simulink model "bus_roadtest_v3"  (R2018a)
settings: Solver=ode3  StartTime=0.0  StopTime=inf  FixedStep=0.01  RelTol=1e-3  EnableMultiTasking=on
PostLoadFcn:
  | , if any(exist('dsrtsu_mdlpostloadfcn', 'file') == [2, 3, 6]), try dsrtsu_mdlpostloadfcn('Execute', bdroot); catch fprintf('Error in PostLoadFcn (dsrtsu_mdlpostloadfcn) for model "%s":\n %s\n', bdroot, lasterr); end, end,
InitFcn:
  | bus_roadtest_v3_initial
values from neighbouring files (symbols this model uses):
  ay_max = 2    [Ini.m]
  delta_t = 0.01    [Ini.m]
  end_left_pass = 1    [Ini.m]
  end_right_pass = 0    [Ini.m]
  finish_node_id = length(Map_data(:,1))    [Ini.m]
  forward_length = 15    [Ini.m]
  gamma = sqrt(N_xaug+lambda)    [bus_roadtest_v3_initial.m]
  k_safe = 1    [Ini.m]
  nodes = nodes(1:index_node,:)    [Ini.m]
  rmin = 10    [Ini.m]
  segments = zeros(length(xy_ends_Pos(:,1)),3)    [Ini.m]
  start_node_id = 1    [Ini.m]
  Ts = 0.01    [bus_roadtest_v3_initial.m]
  Veh_CG = [0.5, 0.2]    [Ini.m]
  Veh_size = [1.99986,6.09558]    [Ini.m]
  vmax = 6    [Ini.m]
  weight = [weight_0,weight_0_cov,weight_i]    [bus_roadtest_v3_initial.m]
undefined symbols (not defined in the file or in its folder): Brake_table, DiscIntNeverNeededParam, Map_data, R, REF_GPS_RFS, Steer_gain_table, T
libraries: rtican x71, simulink x26, rti1401lib_adc_type4 x8, rti1401lib_dio_type4 x1
(part 10 of 18)

== system bus_roadtest_v3/Flag_management/Button management ==
  Button management : MATLAB Function  TreatAsAtomicUnit=on
  Delay3 : Delay  DelayLength=1  InitialCondition=0
  "[Disp] Door1_close_button" : Display
  "[Disp] Door1_open_button" : Display
  "[Disp] Door2_button" : Display
  "[Disp] Door_cmd" : Display
  "[Disp] Door_switch_button" : Display
  "[Disp] Drive_start" : Display
  "[Disp] Drive_start_button" : Display
  "[Disp] Drive_stop" : Display
  "[Disp] Drive_stop_button" : Display
  "[Disp] Emergency_button" : Display
  "[Disp] Emergency_stop" : Display
  "[Disp] PLC_door" : Display
  Drive_start : Outport
  Drive_stop : Outport  Port=2
  Emergency_stop : Outport  Port=3
  Door_cmd : Outport  Port=4
  wires:
  Button management/2(Drive_stop) -> Drive_stop/1, "[Disp] Drive_stop"/1
  Delay3/1 -> Button management/9(Auto_Door)
  Button management/3(Emergency_stop) -> Emergency_stop/1, "[Disp] Emergency_stop"/1
  [Drive_start_button] -> "[Disp] Drive_start_button"/1, Button management/1(Drive_start_button)
  [Door1_open_button] -> "[Disp] Door1_open_button"/1, Button management/5(Door1_open_button)
  Button management/1(Drive_start) -> Drive_start/1, "[Disp] Drive_start"/1
  [Auto_Door] -> Delay3/1
  [Drive_stop_button] -> "[Disp] Drive_stop_button"/1, Button management/2(Drive_stop_button)
  [Door1_close_button] -> "[Disp] Door1_close_button"/1, Button management/6(Door1_close_button)
  [PLC_door] -> "[Disp] PLC_door"/1, Button management/4(Door_state_fb)
  [Emergency_button] -> "[Disp] Emergency_button"/1, Button management/3(Emergency_button)
  [Door_switch_button] -> "[Disp] Door_switch_button"/1, Button management/8(Door_switch_button)
  [Door2_button] -> "[Disp] Door2_button"/1, Button management/7(Door2_button)
  Button management/4(Door_cmd) -> Door_cmd/1, "[Disp] Door_cmd"/1

== system bus_roadtest_v3/Flag_management/Fault detection ==
  Fault detection(Control) : Subsystem
  Fault flags management : MATLAB Function  TreatAsAtomicUnit=on
  "[Disp] Fault_minor" : Display
  "[Disp] Fault_prime" : Display
  Fault_minor : Outport
  Fault_prime : Outport  Port=2
  tag scope: Brake_fault=global, Localization_fault=global, OBU_fault=global, RSU_fault=global, Speed_fault=global, Steer_fault=global
  wires:
  [SLAM_fault] -> Fault flags management/7(SLAM_fault)
  [Speed_fault] -> Fault flags management/3(Speed_fault)
  [OBU_fault] -> Fault flags management/2(OBU_fault)
  [Monitor_fault] -> Fault flags management/1(Monitor_fault)
  [Steer_fault] -> Fault flags management/4(Steer_fault)
  [Brake_fault] -> Fault flags management/5(Brake_fault)
  [RSU_fault] -> Fault flags management/6(RSU_fault)
  Fault detection(Control)/1(Speed_fault) -> [Speed_fault]
  Fault detection(Control)/6(OBU_fault) -> [OBU_fault]
  Fault detection(Control)/5(RSU_fault) -> [RSU_fault]
  Fault detection(Control)/4(SLAM_fault) -> [Localization_fault]
  Fault detection(Control)/3(Brake_fault) -> [Brake_fault]
  Fault detection(Control)/2(Steer_fault) -> [Steer_fault]
  Fault flags management/2(Fault_prime) -> Fault_prime/1, "[Disp] Fault_prime"/1
  Fault flags management/1(Fault_minor) -> Fault_minor/1, "[Disp] Fault_minor"/1

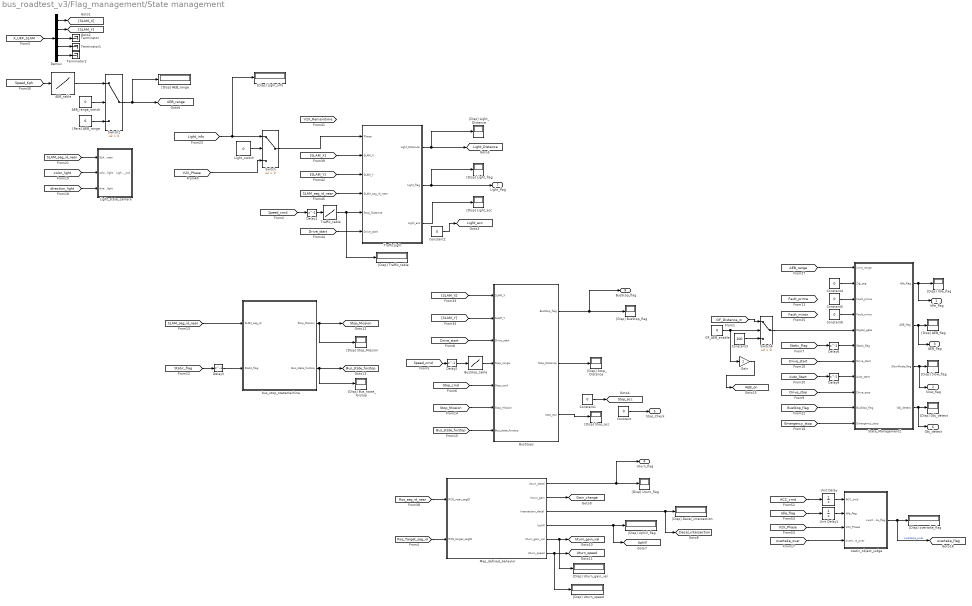
== system bus_roadtest_v3/Flag_management/State management ==
  " BusStops" : MATLAB Function  TreatAsAtomicUnit=on
  AEB_range_switch : Constant  Value=0
  AEB_table : Lookup_n-D  NumberOfTableDimensions=1  BreakpointsForDimension1="[0 5 10 15  20]"  Table=[3 3 4 6 8]  InternalRulePriority=Speed  RndMeth=Simplest  InputSameDT=on
  BusStop_table : Lookup_n-D  NumberOfTableDimensions=1  BreakpointsForDimension1=[0 5 9 13 17]  Table=[4 5.5 11 17 25]  InternalRulePriority=Speed  RndMeth=Simplest  InputSameDT=on
  Constant{,1..2,4..6} (6 alike) : Constant  Value=0
  Constant3 : Constant  Value=100
  Delay{1..3,6,9} (5 alike) : Delay  DelayLength=1  InitialCondition=0
  Demux : Demux  Outputs=5
  GF_AEB_enable : Constant  Value=0
  Gain : Gain
  "Light_state_camera " : MATLAB Function  TreatAsAtomicUnit=on
  Light_switch : Constant  Value=0  VectorParams1D=off  SampleTime=-1
  Map_defined_behavior : MATLAB Function  TreatAsAtomicUnit=on
  State_Management2 : MATLAB Function  TreatAsAtomicUnit=on
  Switch : Switch  Criteria=u2 > Threshold
  Switch2 : Switch  Criteria=u2 > Threshold
  Switch6 : Switch  Criteria=u2 > Threshold
  Terminator : Terminator
  Terminator1 : Terminator
  Terminator2 : Terminator
  TrafficLight : MATLAB Function  TreatAsAtomicUnit=on
  Traffic_table : Lookup_n-D  NumberOfTableDimensions=1  BreakpointsForDimension1=[0 5 9 13 17]  Table=[4 5.5 11 16.5 25]  InternalRulePriority=Speed  RndMeth=Simplest  InputSameDT=on
  Unit Delay : UnitDelay  SampleTime=-1
  Unit Delay1 : UnitDelay  SampleTime=-1
  "[Disp] AEB_flag" : Display
  "[Disp] AEB_range" : Display
  "[Disp] BusStop_flag" : Display
  "[Disp] Bus_state_forstop" : Display
  "[Disp] Decel_intersection" : Display
  "[Disp] Idle_flag" : Display
  "[Disp] Light_Distance" : Display
  "[Disp] Light_acc" : Display
  "[Disp] Light_flag" : Display
  "[Disp] Light_info" : Display
  "[Disp] Obj_detect" : Display
  "[Disp] Slow_flag" : Display
  "[Disp] Stop_Distance" : Display
  "[Disp] Stop_Mission" : Display
  "[Disp] Stop_acc" : Display
  "[Disp] Traffic_table" : Display
  "[Disp] Uphill_flag" : Display
  "[Disp] Uturn_flag" : Display
  "[Disp] Uturn_gain_val" : Display
  "[Disp] Uturn_speed" : Display
  "[Disp] overtake_flag" : Display
  "[Para] AEB_range" : Constant  Value=6
  bus_stop_statemachine : MATLAB Function  TreatAsAtomicUnit=on
  static_object_judge : MATLAB Function  TreatAsAtomicUnit=on
  Idle_flag : Outport
  Slow_flag : Outport  Port=2
  AEB_flag : Outport  Port=3
  Uturn_flag : Outport  Port=4
  Stop_Check : Outport  Port=5
  Obj_detect : Outport  Port=6
  Light_flag : Outport  Port=7
  BusStop_flag : Outport  Port=8
  tag scope: AEB_on=global, AEB_range=global, Bus_state_forstop=global, Decel_intersection=global, Gain_change=global, Light_Distance=global, Light_acc=global, Stop_Mission=global, Stop_acc=global, Uphill=global, Uturn_gain_val=global, Uturn_speed=global, overtake_flag=global
  wires:
  [Static_flag] -> Delay6/1
  Delay6/1 -> State_Management2/6(Static_flag)
  [Drive_stop] -> State_Management2/9(Drive_stop)
  [Drive_start] -> State_Management2/7(Drive_start)
  AEB_table/1 -> Switch2/1
  AEB_range_switch/1 -> Switch2/2
  [Speed_Kph] -> AEB_table/1
  "[Para] AEB_range"/1 -> Switch2/3
  Switch2/1 -> "[Disp] AEB_range"/1, [AEB_range]
  [AEB_range] -> State_Management2/1(Limit_range)
  [X_UKF_SLAM] -> Demux/1
  Demux/5 -> Terminator2/1
  Demux/4 -> Terminator1/1
  Demux/3 -> Terminator/1
  Demux/1 -> [SLAM_X]
  Demux/2 -> [SLAM_Y]
  [SLAM_X] -> " BusStops"/1(SLAM_X)
  [SLAM_Y] -> " BusStops"/2(SLAM_Y)
  [Ros_seg_id_near] -> Map_defined_behavior/1(ROS_near_segID)
  [Drive_start] -> " BusStops"/3(Drive_start)
  [BusStop_flag] -> State_Management2/10(BusStop_flag)
  [SLAM_Y] -> TrafficLight/3(SLAM_Y)
  [SLAM_X] -> TrafficLight/2(SLAM_X)
  [Drive_start] -> TrafficLight/6(Drive_start)
  Map_defined_behavior/1(Uturn_decel) -> Uturn_flag/1, "[Disp] Uturn_flag"/1
  State_Management2/2(AEB_flag) -> AEB_flag/1, "[Disp] AEB_flag"/1
  State_Management2/1(Idle_flag) -> Idle_flag/1, "[Disp] Idle_flag"/1
  State_Management2/4(Obj_detect) -> Obj_detect/1, "[Disp] Obj_detect"/1
  " BusStops"/2(Stop_Distance) -> "[Disp] Stop_Distance"/1
  [SLAM_seg_id_near] -> TrafficLight/4(SLAM_seg_id_near)
  [Auto_Start] -> Delay9/1
  Delay9/1 -> State_Management2/8(Auto_start)
  Constant3/1 -> Switch6/3
  Switch6/1 -> State_Management2/5(Digital_gate)
  GF_AEB_enable/1 -> Gain/1, Switch6/2
  Constant4/1 -> State_Management2/2(Zig_zag)
  Constant5/1 -> State_Management2/3(Fault_prime)
  Constant6/1 -> State_Management2/4(Fault_minor)
  State_Management2/3(SlowMode_flag) -> Slow_flag/1, "[Disp] Slow_flag"/1
  [Emergency_stop] -> State_Management2/11(Emergency_stop)
  TrafficLight/1(Light_Distance) -> "[Disp] Light_Distance"/1, [Light_Distance]
  TrafficLight/2(Light_flag) -> "[Disp] Light_flag"/1, Light_flag/1
  TrafficLight/3(Light_acc) -> "[Disp] Light_acc"/1
  [GF_Distance_m] -> Switch6/1
  [Speed_cmd] -> Delay1/1
  [Ros_Target_seg_id] -> Map_defined_behavior/2(ROS_target_segID)
  Map_defined_behavior/4(Uphill) -> "[Disp] Uphill_flag"/1, [Uphill]
  Map_defined_behavior/3(Intersection_decel) -> [Decel_intersection], "[Disp] Decel_intersection"/1
  Map_defined_behavior/2(Uturn_gain) -> [Gain_change]
  Map_defined_behavior/5(Uturn_gain_val) -> "[Disp] Uturn_gain_val"/1, [Uturn_gain_val]
  Map_defined_behavior/6(Uturn_speed) -> "[Disp] Uturn_speed"/1, [Uturn_speed]
  BusStop_table/1 -> " BusStops"/4(Stop_range)
  [Speed_cmd] -> Delay2/1
  Delay2/1 -> BusStop_table/1
  [Stop_cmd] -> " BusStops"/5(Stop_cmd)
  Delay3/1 -> bus_stop_statemachine/2(Static_flag)
  [Static_flag] -> Delay3/1
  [SLAM_seg_id_near] -> bus_stop_statemachine/1(SLAM_seg_id)
  bus_stop_statemachine/1(Stop_Mission) -> "[Disp] Stop_Mission"/1, [Stop_Mission]
  bus_stop_statemachine/2(Bus_state_forstop) -> "[Disp] Bus_state_forstop"/1, [Bus_state_forstop]
  [Stop_Mission] -> " BusStops"/6(Stop_Mission)
  [Bus_state_forstop] -> " BusStops"/7(Bus_state_forstop)
  Constant/1 -> Stop_Check/1
  " BusStops"/3(stop_acc) -> "[Disp] Stop_acc"/1
  [V2X_Phase] -> static_object_judge/3(V2X_Phase)
  [ACC_cmd] -> Unit Delay/1
  Unit Delay/1 -> static_object_judge/1(ACC_cmd)
  Unit Delay1/1 -> static_object_judge/2(Idle_flag)
  [Idle_flag] -> Unit Delay1/1
  [overtake_over] -> static_object_judge/4(overtake_over)
  Gain/1 -> [AEB_on]
  [color_light] -> "Light_state_camera "/2(color_light)
  [direction_light] -> "Light_state_camera "/3(direction_light)
  [SLAM_seg_id_near] -> "Light_state_camera "/1(SLAM_seg_id_near)
  Light_switch/1 -> Switch/2
  Switch/1 -> TrafficLight/1(Phase)
  [Light_info] -> "[Disp] Light_info"/1, Switch/1
  Delay1/1 -> Traffic_table/1
  Traffic_table/1 -> "[Disp] Traffic_table"/1, TrafficLight/5(Stop_Distance)
  [V2X_Phase] -> Switch/3
  " BusStops"/1(BusStop_flag) -> BusStop_flag/1, "[Disp] BusStop_flag"/1
  Constant1/1 -> [Stop_acc]
  Constant2/1 -> [Light_acc]
  static_object_judge/1(overtake_flag) -> [overtake_flag], "[Disp] overtake_flag"/1  "overtake_over"

== system bus_roadtest_v3/Motion_controller/Lateral_control ==
  Auto_Uturn : Constant
  Gain : Gain  Gain=-180/pi
  Gain1 : Gain  Gain=-1
  LKC_module : Subsystem
  Signal_switch1 : Switch  Criteria=u2 > Threshold
  Signal_switch2 : Switch  Criteria=u2 > Threshold
  Signal_switch3 : Switch  Criteria=u2 > Threshold
  U-turn : Constant  Value=0
  "[Disp] Angle_cmd" : Display
  "[Disp] Auto_Uturn_flag" : Display
  "[Disp] Theta_err" : Display
  "[Disp] Theta_prediction" : Display
  "[Disp] Theta_target" : Display
  "[Para] Look_ahead_Uturn" : Constant  Value=1.6
  "[Para] Look_ahead_time" : Constant  Value=1.6
  tag scope: Steer_cmd=global, U_turn=global
  wires:
  [SBG_Gyro_Z] -> Gain/1
  LKC_module/2(Theta_prediction) -> "[Disp] Theta_prediction"/1
  LKC_module/3(Theta_err) -> "[Disp] Theta_err"/1
  LKC_module/4(Theta_target) -> "[Disp] Theta_target"/1
  [Speed_mps] -> LKC_module/3(Vx)
  LKC_module/1(Steerwheel_cmd) -> [Steer_cmd], "[Disp] Angle_cmd"/1
  [Look_ahead_S0] -> LKC_module/2(Look_ahead_S0)
  Signal_switch1/1 -> LKC_module/1(Look_ahead_time)
  "[Para] Look_ahead_time"/1 -> Signal_switch1/3
  "[Para] Look_ahead_Uturn"/1 -> Signal_switch1/1
  Signal_switch2/1 -> Signal_switch1/2, [U_turn]
  U-turn/1 -> Signal_switch2/3
  Auto_Uturn/1 -> Signal_switch2/2
  [angular_vz] -> Gain1/1
  Gain1/1 -> LKC_module/5(yaw_rate_IMU)
  [Gain_change] -> "[Disp] Auto_Uturn_flag"/1, Signal_switch3/2, Signal_switch2/1
  Signal_switch3/1 -> LKC_module/4(Y_target)
  [Ros_rear_Vehicle_Target_y] -> Signal_switch3/3
  [Ros_Vehicle_Target_y] -> Signal_switch3/1

== system bus_roadtest_v3/Motion_controller/Longitudinal_control ==
  Speed_profile : Inport
  AEB_trig : Inport  Port=2
  Static : Inport  Port=3
  Brake_controller : Subsystem
  Data Type Conversion : DataTypeConversion  OutDataTypeStr=boolean
  Fbrake_Pcmd : Constant  Value=0
  Fbrake_mode : Constant
  Memory : Memory
  Rbrake_Pcmd : Constant  Value=0
  Rbrake_mode : Constant
  Switching_module : Subsystem
  Throttle_controller : Subsystem
  Throttle_mode : Constant
  Throttle_vol : Constant  Value=0
  "[Disp] Fbrake_Vcmd" : Display
  "[Disp] Rbrake_Vcmd" : Display
  "[Disp] Throttle_Vcmd" : Display
  tag scope: Fbrake_Vcmd=global, Rbrake_Vcmd=global, Throttle_Vcmd=global
  wires:
  Speed_profile/1 -> Brake_controller/9(Speed_profile), Switching_module/3(Speed_profile)
  Switching_module/3(Brake_trig_CC) -> Memory/1, Brake_controller/8(Brake_trig_CC)
  Memory/1 -> Data Type Conversion/1
  Throttle_mode/1 -> Throttle_controller/1(Throttle_mode)
  Throttle_vol/1 -> Throttle_controller/2(Throttle_vol)
  Throttle_controller/1(Throttle_out) -> "[Disp] Throttle_Vcmd"/1, [Throttle_Vcmd]
  AEB_trig/1 -> Switching_module/1(AEB_trig), Brake_controller/1(AEB_trig), Throttle_controller/3(AEB_trig)
  Static/1 -> Switching_module/2(Static), Brake_controller/2(Static), Throttle_controller/4(Static)
  Fbrake_mode/1 -> Brake_controller/4(Fbrake_mode)
  Fbrake_Pcmd/1 -> Brake_controller/5(Fbrake_Pcmd)
  Brake_controller/1(Fbrake_Vcmd) -> "[Disp] Fbrake_Vcmd"/1, [Fbrake_Vcmd]
  Data Type Conversion/1 -> Switching_module/4(Brake_trig_CC_status)
  Switching_module/1(Speed_cmd) -> Throttle_controller/5(Speed_cmd)
  Switching_module/2(Decel_cmd) -> Brake_controller/3(Decel_cmd)
  Rbrake_Pcmd/1 -> Brake_controller/7(Rbrake_Pcmd)
  Rbrake_mode/1 -> Brake_controller/6(Rbrake_mode)
  Brake_controller/2(Rbrake_Vcmd) -> "[Disp] Rbrake_Vcmd"/1, [Rbrake_Vcmd]

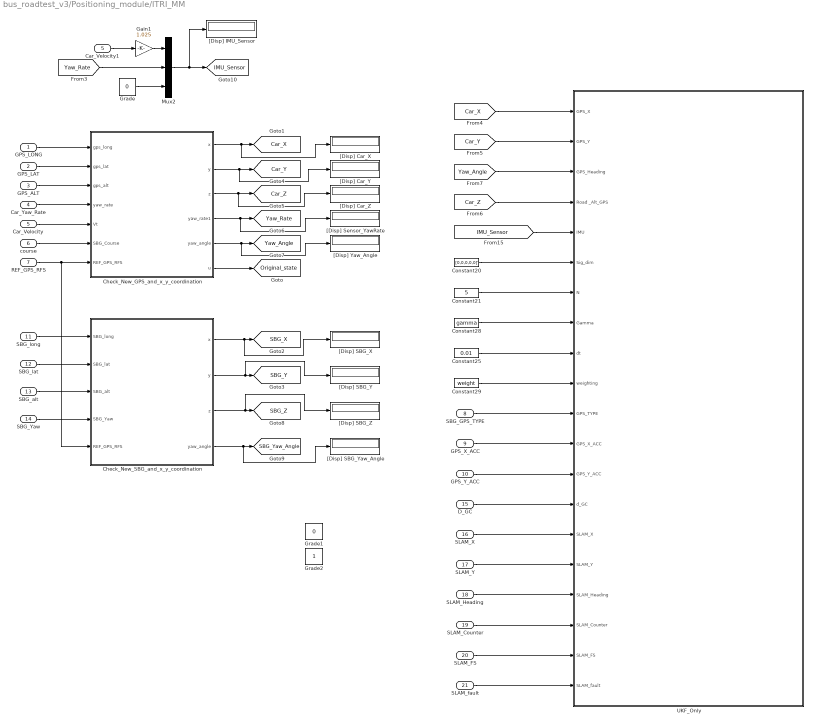
== system bus_roadtest_v3/Positioning_module/ITRI_MM ==
  GPS_LONG : Inport
  GPS_LAT : Inport  Port=2
  GPS_ALT : Inport  Port=3
  Car_Yaw_Rate : Inport  Port=4
  Car_Velocity : Inport  Port=5
  course : Inport  Port=6
  REF_GPS_RFS : Inport  Port=7
  SBG_GPS_TYPE : Inport  Port=8
  GPS_X_ACC : Inport  Port=9
  GPS_Y_ACC : Inport  Port=10
  SBG_long : Inport  Port=11
  SBG_lat : Inport  Port=12
  SBG_alt : Inport  Port=13
  SBG_Yaw : Inport  Port=14
  D_GC : Inport  Port=15
  SLAM_X : Inport  Port=16
  SLAM_Y : Inport  Port=17
  SLAM_Heading : Inport  Port=18
  SLAM_Counter : Inport  Port=19
  SLAM_FS : Inport  Port=20
  SLAM_fault : Inport  Port=21
  Car_Velocity1 : InportShadow  Port=5
  Check_New_GPS_and_x_y_coordination : MATLAB Function  TreatAsAtomicUnit=on
  Check_New_SBG_and_x_y_coordination : MATLAB Function  TreatAsAtomicUnit=on
  Constant20 : Constant  Value=[0,0,0,0,0]'
  Constant21 : Constant  Value=5
  Constant25 : Constant  Value=0.01
  Constant28 : Constant  Value=gamma
  Constant29 : Constant  Value=weight
  Gain1 : Gain  Gain=1.025
  Grade : Constant  Value=0
  Grade1 : Constant  Value=0
  Grade2 : Constant
  Mux2 : Mux  Inputs=3
  UKF_Only : Subsystem
  "[Disp] Car_X" : Display
  "[Disp] Car_Y" : Display
  "[Disp] Car_Z" : Display
  "[Disp] IMU_Sensor" : Display
  "[Disp] SBG_X" : Display
  "[Disp] SBG_Y" : Display
  "[Disp] SBG_Yaw_Angle" : Display
  "[Disp] SBG_Z" : Display
  "[Disp] Sensor_YawRate" : Display
  "[Disp] Yaw_Angle" : Display
  tag scope: Car_X=global, Car_Y=global, Car_Z=global, IMU_Sensor=global, Original_state=global, SBG_X=global, SBG_Y=global, SBG_Yaw_Angle=global, SBG_Z=global, Yaw_Angle=global, Yaw_Rate=global
  wires:
  GPS_LONG/1 -> Check_New_GPS_and_x_y_coordination/1(gps_long)
  GPS_LAT/1 -> Check_New_GPS_and_x_y_coordination/2(gps_lat)
  GPS_ALT/1 -> Check_New_GPS_and_x_y_coordination/3(gps_alt)
  Car_Yaw_Rate/1 -> Check_New_GPS_and_x_y_coordination/4(yaw_rate)
  Car_Velocity/1 -> Check_New_GPS_and_x_y_coordination/5(Vt)
  Check_New_GPS_and_x_y_coordination/1(x) -> "[Disp] Car_X"/1, [Car_X]
  REF_GPS_RFS/1 -> Check_New_SBG_and_x_y_coordination/5(REF_GPS_RFS), Check_New_GPS_and_x_y_coordination/7(REF_GPS_RFS)
  Car_Velocity1/1 -> Gain1/1
  Mux2/1 -> "[Disp] IMU_Sensor"/1, [IMU_Sensor]
  Gain1/1 -> Mux2/1
  [IMU_Sensor] -> UKF_Only/5(IMU)
  Constant20/1 -> UKF_Only/6(Sig_dim)
  Constant21/1 -> UKF_Only/7(N)
  Constant28/1 -> UKF_Only/8(Gamma)
  Constant25/1 -> UKF_Only/9(dt)
  Constant29/1 -> UKF_Only/10(weighting)
  [Yaw_Angle] -> UKF_Only/3(GPS_Heading)
  Check_New_GPS_and_x_y_coordination/6(u) -> [Original_state]
  Check_New_GPS_and_x_y_coordination/2(y) -> "[Disp] Car_Y"/1, [Car_Y]
  Check_New_GPS_and_x_y_coordination/3(z) -> "[Disp] Car_Z"/1, [Car_Z]
  Check_New_GPS_and_x_y_coordination/4(yaw_rate1) -> "[Disp] Sensor_YawRate"/1, [Yaw_Rate]
  [Car_Z] -> UKF_Only/4(Road _Alt_GPS)
  Check_New_GPS_and_x_y_coordination/5(yaw_angle) -> "[Disp] Yaw_Angle"/1, [Yaw_Angle]
  course/1 -> Check_New_GPS_and_x_y_coordination/6(SBG_Course)
  Grade/1 -> Mux2/3
  [Car_X] -> UKF_Only/1(GPS_X)
  [Car_Y] -> UKF_Only/2(GPS_Y)
  [Yaw_Rate] -> Mux2/2
  SBG_GPS_TYPE/1 -> UKF_Only/11(GPS_TYPE)
  GPS_X_ACC/1 -> UKF_Only/12(GPS_X_ACC)
  GPS_Y_ACC/1 -> UKF_Only/13(GPS_Y_ACC)
  SBG_long/1 -> Check_New_SBG_and_x_y_coordination/1(SBG_long)
  SBG_lat/1 -> Check_New_SBG_and_x_y_coordination/2(SBG_lat)
  SBG_alt/1 -> Check_New_SBG_and_x_y_coordination/3(SBG_alt)
  SBG_Yaw/1 -> Check_New_SBG_and_x_y_coordination/4(SBG_Yaw)
  Check_New_SBG_and_x_y_coordination/1(x) -> "[Disp] SBG_X"/1, [SBG_X]
  Check_New_SBG_and_x_y_coordination/2(y) -> "[Disp] SBG_Y"/1, [SBG_Y]
  Check_New_SBG_and_x_y_coordination/3(z) -> "[Disp] SBG_Z"/1, [SBG_Z]
  Check_New_SBG_and_x_y_coordination/4(yaw_angle) -> "[Disp] SBG_Yaw_Angle"/1, [SBG_Yaw_Angle]
  D_GC/1 -> UKF_Only/14(d_GC)
  SLAM_X/1 -> UKF_Only/15(SLAM_X)
  SLAM_Y/1 -> UKF_Only/16(SLAM_Y)
  SLAM_Heading/1 -> UKF_Only/17(SLAM_Heading)
  SLAM_Counter/1 -> UKF_Only/18(SLAM_Counter)
  SLAM_FS/1 -> UKF_Only/19(SLAM_FS)
  SLAM_fault/1 -> UKF_Only/20(SLAM_fault)

== system bus_roadtest_v3/RTI Data/RTI Data Store ==
  RTI Data Store : Subsystem  mask(RTI_DATA_STORE){}
      mask help:
      | RTI Data Store Block. This block is used by RTI to store internal model dependent data. Deleting this block will result in data loss.
      |
      | NEVER DELETE, COPY, OR MODIFY THIS BLOCK!
      mask Help:
      | RTI Data Store Block. This block is used by RTI to store internal model dependent data. Deleting this block will result in data loss.
      | 
      | NEVER DELETE, COPY, OR MODIFY THIS BLOCK!
      mask Display: text(0.5, 0.5, ' ', 'HorizontalAlignment', 'center');

== system bus_roadtest_v3/Speed_profile/Auto & Check ==
  Auto_Door : MATLAB Function  TreatAsAtomicUnit=on
  Auto_start : MATLAB Function  TreatAsAtomicUnit=on
  Delay : Delay  DelayLength=1  InitialCondition=0
  Delay2 : Delay  DelayLength=1  InitialCondition=0
  Delay3 : Delay  DelayLength=1  InitialCondition=0
  Static_check : MATLAB Function  TreatAsAtomicUnit=on
  "[Disp] AEBOn" : Display
  "[Disp] AEBStatic" : Display
  "[Disp] AEB_count" : Display
  "[Disp] Auto_Door" : Display
  "[Disp] Auto_Start" : Display
  "[Disp] Door_count" : Display
  "[Disp] Static_flag" : Display
  Static_flag : Outport
  "Auto_Door " : Outport  Port=2
  Auto_Start : Outport  Port=3
  wires:
  Static_check/1(Static_flag) -> Static_flag/1, "[Disp] Static_flag"/1
  [Speed_cmd] -> Delay2/1
  [Speed_Kph] -> Static_check/2(Speed_fb)
  Delay3/1 -> Auto_start/6(Static_flag)
  [Static_flag] -> Auto_Door/1(Static_flag)
  [Throttle_Vcmd] -> Delay/1
  [Stop_Check] -> Auto_start/1(Stop_Check)
  Auto_Door/1(Auto_Door) -> "Auto_Door "/1, "[Disp] Auto_Door"/1
  [Static_flag] -> Delay3/1
  [Stop_Check] -> Auto_Door/2(Stop_Check)
  [Drive_stop] -> Auto_start/4(Drive_stop)
  Delay2/1 -> Static_check/1(Speed_cmd)
  Auto_start/4(AEBOn) -> "[Disp] AEBOn"/1
  Auto_Door/2(Door_count) -> "[Disp] Door_count"/1
  [Drive_start] -> Auto_start/5(Drive_start)
  [Obj_detect] -> Auto_start/2(Obj_detect)
  Delay/1 -> Static_check/3(Throttle_cmd)
  Auto_start/3(AEBStatic) -> "[Disp] AEBStatic"/1
  Auto_start/2(AEB_count) -> "[Disp] AEB_count"/1
  Auto_start/1(AutoStart) -> Auto_Start/1, "[Disp] Auto_Start"/1
  [Emergency_stop] -> Auto_start/3(Emergency_stop)

== system bus_roadtest_v3/Speed_profile/High level controller ==
  ACC : Subsystem
  Add1 : Sum
  Constant{,1..3} (4 alike) : Constant  Value=0
  Constant4 : Constant  Value=1000
  Constant5 : Constant  Value=1000
  Dec_gain : Gain  Gain=0.03
  Delay2 : Delay  DelayLength=1  InitialCondition=0
  Delay3 : Delay  DelayLength=1  InitialCondition=0
  Gain : Gain
  Min : MinMax  Inputs=3
  Relational Operator : RelationalOperator  Operator=<  OutDataTypeStr=boolean  RndMeth=Simplest
  Sample_time1 : Constant  Value=Ts
  SpeedProfile : MATLAB Function  TreatAsAtomicUnit=on
  Switch{,1..3,5} (5 alike) : Switch  Criteria=u2 > Threshold
  "[Disp] Deceleration" : Scope
  "[Disp] New_ACC" : Display
  "[Disp] Speed_cmd" : Display
  "[Disp] Speed_desire" : Display
  "[Disp] Speed_set" : Display
  "[Para] ACC_switch" : Constant  Value=0
  "[Para] Acceleration_cons" : Constant  Value=0.25
  "[Para] Deceleration_cons" : Constant  Value=0.3
  "[Para] Speed_setting" : Constant  Value=10
  "[Para] Uphill_speed" : Constant  Value=17
  "[Para]PP_enable" : Constant  Value=0
  "ccc " : Constant  Value=0
  Speed_cmd : Outport
  tag scope: ACC_cmd=global, ACC_on=global
  wires:
  [Idle_flag] -> SpeedProfile/5(Idle_flag)
  [AEB_flag] -> SpeedProfile/6(AEB_flag)
  [Light_flag] -> SpeedProfile/7(Light_flag)
  Sample_time1/1 -> SpeedProfile/11(Delta_t)
  [Speed_cmd] -> Delay3/1
  SpeedProfile/1(Speed_cmd) -> Speed_cmd/1, "[Disp] Speed_cmd"/1
  SpeedProfile/2(Speed_desire) -> "[Disp] Speed_desire"/1
  Delay3/1 -> SpeedProfile/12(Speed_fb)
  "[Para] Acceleration_cons"/1 -> SpeedProfile/4(Acceleration_cons)
  "[Para] Deceleration_cons"/1 -> Add1/1
  [Speed_cmd] -> Delay2/1
  Dec_gain/1 -> Add1/2
  Delay2/1 -> Dec_gain/1
  Add1/1 -> [Deceleration], "[Disp] Deceleration"/1
  [Deceleration] -> SpeedProfile/3(Deceleration_cons)
  Switch1/1 -> [ACC_cmd], "[Disp] Speed_set"/1
  [Speed_set] -> SpeedProfile/14(Speed_set)
  [Speed_Kph] -> ACC/1(Ego_speed)
  "[Para] ACC_switch"/1 -> Gain/1, Switch1/2
  ACC/1(Speed_cmd) -> Switch1/1, "[Disp] New_ACC"/1
  ACC/2(close_flag) -> [close_flag]
  [PPGF_Stop] -> Switch/1
  Constant2/1 -> Switch/2, Switch/3
  [GF_Distance_m] -> Relational Operator/2, Min/1
  [Uturn_speed] -> SpeedProfile/13(Uturn_speed)
  [ACC_cmd] -> SpeedProfile/16(ACC_cmd)
  Switch2/1 -> Switch1/3, ACC/4(Speed_set), [Speed_set]
  "[Para] Speed_setting"/1 -> Switch2/3
  "[Para] Uphill_speed"/1 -> Switch2/1
  [overtake_flag] -> SpeedProfile/10(overtake_flag)
  Gain/1 -> [ACC_on]
  Constant3/1 -> SpeedProfile/9(Slow_flag)
  [Uturn_flag] -> SpeedProfile/8(Uturn_flag)
  [Light_acc] -> SpeedProfile/1(Light_zone)
  [Stop_acc] -> SpeedProfile/2(Stop_zone)
  [Uphill] -> Switch2/2
  [PPGF_distance] -> Switch3/1
  Constant4/1 -> Switch3/3
  Switch3/1 -> Min/2
  Min/1 -> ACC/3(Rel_distance), Relational Operator/1
  Switch5/1 -> ACC/2(Front_abs_speed)
  [GF_Speed_ms] -> Switch5/3
  Constant/1 -> Switch5/1
  Relational Operator/1 -> Switch5/2
  Switch/1 -> SpeedProfile/15(PPGF_Stop)
  Constant5/1 -> Min/3
  "[Para]PP_enable"/1 -> Switch3/2

== system bus_roadtest_v3/Target_planner/Enabled Subsystem ==
  nodes : Inport
  segrments : Inport  Port=2
  start_id : Inport  Port=3
  finish_id : Inport  Port=4
  Enable : EnablePort  PropagateVarSize=During execution
  Dijkstra : MATLAB Function  TreatAsAtomicUnit=on
  dist : Outport
  path : Outport  Port=2
  nn : Outport  Port=3
  wires:
  nodes/1 -> Dijkstra/1(nodes)
  segrments/1 -> Dijkstra/2(segments)
  start_id/1 -> Dijkstra/3(start_id)
  finish_id/1 -> Dijkstra/4(finish_id)
  Dijkstra/2(path_2) -> path/1
  Dijkstra/1(dist) -> dist/1
  Dijkstra/3(nn) -> nn/1

== system bus_roadtest_v3/Data_RX/Control_button/Push_button1 ==
  Pin_input : Inport
  ADC_gain : Gain  Gain=20
  Compare To Constant : simulink/Logic and Bit Operations/Compare To Constant  relop=<=  const=3.6  OutDataTypeStr=boolean
  Logical Operator : Logic  Operator=NAND  AllPortsSameDT=off  OutDataTypeStr=boolean
  Logical Operator1 : Logic  Operator=NOT  AllPortsSameDT=off  OutDataTypeStr=boolean
  Logical Operator2 : Logic  Operator=NAND  AllPortsSameDT=off  OutDataTypeStr=boolean
  Operation_gain : Gain  Gain=3
  Sum : Sum  Inputs=|+-
  Unit Delay2 : UnitDelay  InitialCondition=1  SampleTime=-1
  Rising_edge : Outport
  Falling_edge : Outport  Port=2
  wires:
  ADC_gain/1 -> Operation_gain/1
  Sum/1 -> ADC_gain/1
  Operation_gain/1 -> Compare To Constant/1
  Logical Operator1/1 -> Logical Operator/2
  Compare To Constant/1 -> Logical Operator1/1, Logical Operator2/1
  Logical Operator2/1 -> Unit Delay2/1, Rising_edge/1
  Logical Operator/1 -> Falling_edge/1, Logical Operator2/2
  Unit Delay2/1 -> Logical Operator/1
  Pin_input/1 -> Sum/1

== system bus_roadtest_v3/Data_RX/Control_button/Push_button2 ==
  Pin_input : Inport
  ADC_gain : Gain  Gain=20
  Compare To Constant : simulink/Logic and Bit Operations/Compare To Constant  relop=<=  const=3.6  OutDataTypeStr=boolean
  Logical Operator : Logic  Operator=NAND  AllPortsSameDT=off  OutDataTypeStr=boolean
  Logical Operator1 : Logic  Operator=NOT  AllPortsSameDT=off  OutDataTypeStr=boolean
  Logical Operator2 : Logic  Operator=NAND  AllPortsSameDT=off  OutDataTypeStr=boolean
  Operation_gain : Gain  Gain=3
  Sum : Sum  Inputs=|+-
  Unit Delay2 : UnitDelay  InitialCondition=1  SampleTime=-1
  Rising_edge : Outport
  Falling_edge : Outport  Port=2
  wires:
  ADC_gain/1 -> Operation_gain/1
  Sum/1 -> ADC_gain/1
  Operation_gain/1 -> Compare To Constant/1
  Logical Operator1/1 -> Logical Operator/2
  Compare To Constant/1 -> Logical Operator1/1, Logical Operator2/1
  Logical Operator2/1 -> Unit Delay2/1, Rising_edge/1
  Logical Operator/1 -> Falling_edge/1, Logical Operator2/2
  Unit Delay2/1 -> Logical Operator/1
  Pin_input/1 -> Sum/1

== system bus_roadtest_v3/Data_RX/Control_button/Push_button4 ==
  Pin_input : Inport
  ADC_gain : Gain  Gain=20
  Compare To Constant : simulink/Logic and Bit Operations/Compare To Constant  relop=<=  const=3.6  OutDataTypeStr=boolean
  Logical Operator : Logic  Operator=NAND  AllPortsSameDT=off  OutDataTypeStr=boolean
  Logical Operator1 : Logic  Operator=NOT  AllPortsSameDT=off  OutDataTypeStr=boolean
  Logical Operator2 : Logic  Operator=NAND  AllPortsSameDT=off  OutDataTypeStr=boolean
  Operation_gain : Gain  Gain=3
  Sum : Sum  Inputs=|+-
  Unit Delay2 : UnitDelay  InitialCondition=1  SampleTime=-1
  Rising_edge : Outport
  Falling_edge : Outport  Port=2
  wires:
  ADC_gain/1 -> Operation_gain/1
  Sum/1 -> ADC_gain/1
  Operation_gain/1 -> Compare To Constant/1
  Logical Operator1/1 -> Logical Operator/2
  Compare To Constant/1 -> Logical Operator1/1, Logical Operator2/1
  Logical Operator2/1 -> Unit Delay2/1, Rising_edge/1
  Logical Operator/1 -> Falling_edge/1, Logical Operator2/2
  Unit Delay2/1 -> Logical Operator/1
  Pin_input/1 -> Sum/1

== system bus_roadtest_v3/Data_RX/Control_button/Push_button5 ==
  Pin_input : Inport
  ADC_gain : Gain  Gain=20
  Compare To Constant : simulink/Logic and Bit Operations/Compare To Constant  relop=<=  const=3.6  OutDataTypeStr=boolean
  Logical Operator : Logic  Operator=NAND  AllPortsSameDT=off  OutDataTypeStr=boolean
  Logical Operator1 : Logic  Operator=NOT  AllPortsSameDT=off  OutDataTypeStr=boolean
  Logical Operator2 : Logic  Operator=NAND  AllPortsSameDT=off  OutDataTypeStr=boolean
  Operation_gain : Gain  Gain=3
  Sum : Sum  Inputs=|+-
  Unit Delay2 : UnitDelay  InitialCondition=1  SampleTime=-1
  Rising_edge : Outport
  Falling_edge : Outport  Port=2
  wires:
  ADC_gain/1 -> Operation_gain/1
  Sum/1 -> ADC_gain/1
  Operation_gain/1 -> Compare To Constant/1
  Logical Operator1/1 -> Logical Operator/2
  Compare To Constant/1 -> Logical Operator1/1, Logical Operator2/1
  Logical Operator2/1 -> Unit Delay2/1, Rising_edge/1
  Logical Operator/1 -> Falling_edge/1, Logical Operator2/2
  Unit Delay2/1 -> Logical Operator/1
  Pin_input/1 -> Sum/1

== system bus_roadtest_v3/Data_RX/Control_button/Push_button6 ==
  Pin_input : Inport
  ADC_gain : Gain  Gain=20
  Compare To Constant : simulink/Logic and Bit Operations/Compare To Constant  relop=<=  const=3.6  OutDataTypeStr=boolean
  Logical Operator : Logic  Operator=NAND  AllPortsSameDT=off  OutDataTypeStr=boolean
  Logical Operator1 : Logic  Operator=NOT  AllPortsSameDT=off  OutDataTypeStr=boolean
  Logical Operator2 : Logic  Operator=NAND  AllPortsSameDT=off  OutDataTypeStr=boolean
  Operation_gain : Gain  Gain=3
  Sum : Sum  Inputs=|+-
  Unit Delay2 : UnitDelay  InitialCondition=1  SampleTime=-1
  Rising_edge : Outport
  Falling_edge : Outport  Port=2
  wires:
  ADC_gain/1 -> Operation_gain/1
  Sum/1 -> ADC_gain/1
  Operation_gain/1 -> Compare To Constant/1
  Logical Operator1/1 -> Logical Operator/2
  Compare To Constant/1 -> Logical Operator1/1, Logical Operator2/1
  Logical Operator2/1 -> Unit Delay2/1, Rising_edge/1
  Logical Operator/1 -> Falling_edge/1, Logical Operator2/2
  Unit Delay2/1 -> Logical Operator/1
  Pin_input/1 -> Sum/1

== system bus_roadtest_v3/Data_RX/Control_button/Push_button7 ==
  Pin_input : Inport
  ADC_gain : Gain  Gain=20
  Compare To Constant : simulink/Logic and Bit Operations/Compare To Constant  relop=<=  const=3.6  OutDataTypeStr=boolean
  Logical Operator : Logic  Operator=NAND  AllPortsSameDT=off  OutDataTypeStr=boolean
  Logical Operator1 : Logic  Operator=NOT  AllPortsSameDT=off  OutDataTypeStr=boolean
  Logical Operator2 : Logic  Operator=NAND  AllPortsSameDT=off  OutDataTypeStr=boolean
  Operation_gain : Gain  Gain=3
  Sum : Sum  Inputs=|+-
  Unit Delay2 : UnitDelay  InitialCondition=1  SampleTime=-1
  Rising_edge : Outport
  Falling_edge : Outport  Port=2
  wires:
  ADC_gain/1 -> Operation_gain/1
  Sum/1 -> ADC_gain/1
  Operation_gain/1 -> Compare To Constant/1
  Logical Operator1/1 -> Logical Operator/2
  Compare To Constant/1 -> Logical Operator1/1, Logical Operator2/1
  Logical Operator2/1 -> Unit Delay2/1, Rising_edge/1
  Logical Operator/1 -> Falling_edge/1, Logical Operator2/2
  Unit Delay2/1 -> Logical Operator/1
  Pin_input/1 -> Sum/1

== system bus_roadtest_v3/Data_RX/Control_button/Toggle_Motor_Driver ==
  Pin_input : Inport
  ADC_gain : Gain  Gain=20
  Compare To Constant : simulink/Logic and Bit Operations/Compare To Constant  relop=<=  const=2.4  OutDataTypeStr=boolean
  Operation_gain : Gain  Gain=3
  Sum : Sum  Inputs=|+-
  Switch_on : Outport
  wires:
  Pin_input/1 -> Sum/1
  Compare To Constant/1 -> Switch_on/1
  ADC_gain/1 -> Operation_gain/1
  Sum/1 -> ADC_gain/1
  Operation_gain/1 -> Compare To Constant/1

== system bus_roadtest_v3/Data_RX/Control_button/Toggle_Motor_Driver1 ==
  Pin_input : Inport
  ADC_gain : Gain  Gain=20
  Compare To Constant : simulink/Logic and Bit Operations/Compare To Constant  relop=<=  const=3.6  OutDataTypeStr=boolean
  Operation_gain : Gain  Gain=3
  Sum : Sum  Inputs=|+-
  Switch_on : Outport
  wires:
  Pin_input/1 -> Sum/1
  Compare To Constant/1 -> Switch_on/1
  ADC_gain/1 -> Operation_gain/1
  Sum/1 -> ADC_gain/1
  Operation_gain/1 -> Compare To Constant/1
